simulink model "blockdemo"  (Simulink 6.3)
settings: Solver=ode45  StartTime=0.0  StopTime=10.0  RelTol=1e-3
InitFcn:
  | %% DSPBuilder Start
  | alt_dspbuilder_update_model(bdroot)
  | %% DSPBuilder End
libraries: allblocks_alteradspbuilder2 x12
settings Model: Creator=cpurcell  LastModifiedBy=delphick
settings DebuggingCC: MultiTaskDSMMsg=error

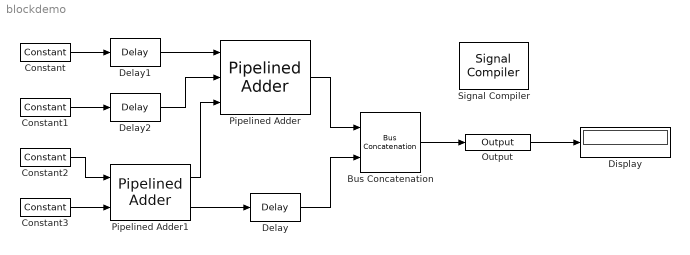
== system blockdemo ==
  Bus Concatenation : allblocks_alteradspbuilder2/Bus Concatenation  isSigned=on  awidth=9  bwidth=9
  Constant : allblocks_alteradspbuilder2/Constant  mask_cst=5  BusType=Signed Integer  bwl=8  bwr=0  SpecifyClock=off
  Constant1 : allblocks_alteradspbuilder2/Constant  mask_cst=-8  BusType=Signed Integer  bwl=8  bwr=0  SpecifyClock=off
  Constant2 : allblocks_alteradspbuilder2/Constant  mask_cst=28  BusType=Unsigned Integer  bwl=8  bwr=0  SpecifyClock=off
  Constant3 : allblocks_alteradspbuilder2/Constant  mask_cst=33  BusType=Unsigned Integer  bwl=8  bwr=0  SpecifyClock=off
  Delay : allblocks_alteradspbuilder2/Delay  pipeline=1  ClockPhase=1  use_ena=off  use_sclr=off
  Delay1 : allblocks_alteradspbuilder2/Delay  pipeline=1  ClockPhase=1  use_ena=off  use_sclr=off
  Delay2 : allblocks_alteradspbuilder2/Delay  pipeline=1  ClockPhase=1  use_ena=off  use_sclr=off
  Display : Display
  Output : allblocks_alteradspbuilder2/Output  iofile=C:\workspace_clean\Documentation\DesignExamples\Tutorials\UnitBlocks\Arithmetic\PipelinedAdder\tb_blockdemo\blockdemo_Output.capture  BusType=Inferred  bwl=8  bwr=0  PORTTYPE=Output
  Pipelined Adder : allblocks_alteradspbuilder2/Pipelined Adder  BusType=Signed Integer  bwl=8  bwr=0  pipeline=1  AddSubDirection=ADD  use_cin=on  use_ovl=off  use_addsub=off  use_ena=off  use_aclr=off
  Pipelined Adder1 : allblocks_alteradspbuilder2/Pipelined Adder  BusType=Unsigned Integer  bwl=8  bwr=0  pipeline=1  AddSubDirection=ADD  use_cin=off  use_ovl=on  use_addsub=off  use_ena=off  use_aclr=off
  Signal Compiler : allblocks_alteradspbuilder2/Signal Compiler  DeviceFamily=Stratix IV  DeviceName=AUTO  EnableSignalTap=off  SignalTapDepth=128  UseBoardBlock=off  StpUseDefaultClock=on  StpClock=clock
  wires:
  Pipelined Adder1/1 -> Pipelined Adder/3
  Delay1/1 -> Pipelined Adder/1
  Delay2/1 -> Pipelined Adder/2
  Pipelined Adder1/2 -> Delay/1
  Pipelined Adder/1 -> Bus Concatenation/1
  Delay/1 -> Bus Concatenation/2
  Constant/1 -> Delay1/1
  Constant1/1 -> Delay2/1
  Constant2/1 -> Pipelined Adder1/1
  Constant3/1 -> Pipelined Adder1/2
  Bus Concatenation/1 -> Output/1
  Output/1 -> Display/1
